simulink model "Record_Test"  (R2020a)
settings: Solver=VariableStepAuto  StartTime=0.0  StopTime=10  RelTol=1e-3
libraries: dspstat3 x3, audiosources x1, simulink x1, dspfdesign x1, dspvision x1, audiomeasurements x1
settings Model: Creator=Emil  LastModifiedBy=Emil

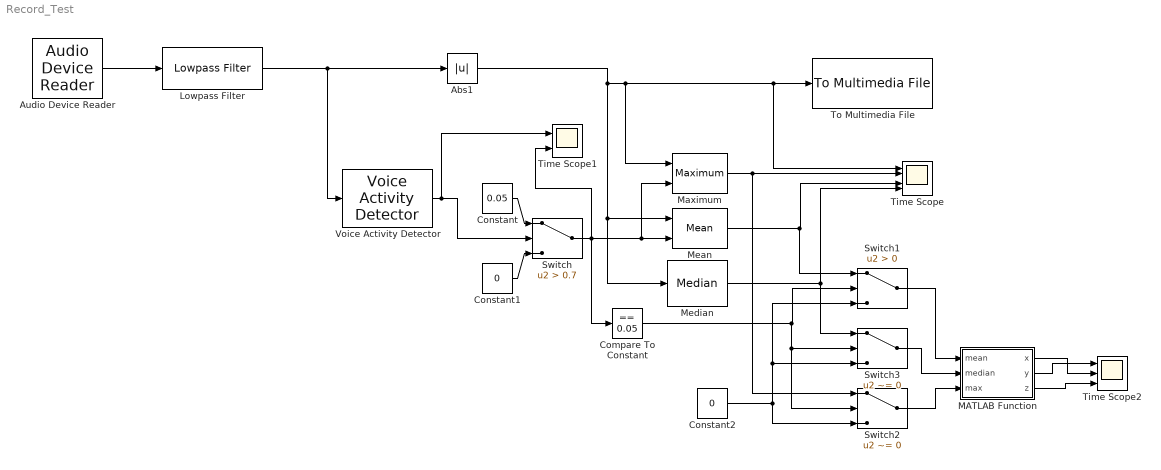
== system Record_Test ==
  Abs1 : Abs
  Audio Device Reader : audiosources/Audio Device Reader  Driver=DirectSound  Device=Default  SampleRate=44100  NumChannels=1  SamplesPerFrame=1024  BitDepth=16-bit integer  NumBuffers=10  DefaultInputChannelMapping=on  InputChannelMapping=1:2  OutputNumOverrunSamples=off  OutputDataType=double  DriverIdx=1  DeviceWarnFlag=''
      settings: SourceProductBaseCode=AU
  Compare To Constant : simulink/Logic and Bit Operations/Compare To Constant  relop===  const=0.05  OutDataTypeStr=boolean
  Constant : Constant  Value=0.05
  Constant1 : Constant  Value=0
  Constant2 : Constant  Value=0
  Lowpass Filter : dspfdesign/Lowpass Filter  FilterType=FIR  DesignForMinimumOrder=on  FilterOrder=50  PassbandFrequency=2.2e3  StopbandFrequency=3e3  PassbandRipple=0.1  StopbandAttenuation=80  InheritSampleRate=off  SampleRate=44100  SimulateUsing=Interpreted execution  roundingMode=Floor  coeffsDataTypeStr=fixdt(1,16)
  MATLAB Function : MATLAB Function  TreatAsAtomicUnit=on
  Maximum : dspstat3/Maximum  operation=maximum  fcn=Running  indexBase=One  operateOver=Entire input  Dimension=1  InputProcessing=Columns as channels (frame based)  reset=Either edge  roiEnable=off  roiType=Rectangles  roiPortion=Entire ROI  roiOutput=Individual statistics for each ROI  roiFlag=off  roundingMode=Nearest  overflowMode=off  accumDataTypeStr=Inherit: Same as product output  accumLastDataTypeStr=Inherit: Same as product output
  Mean : dspstat3/Mean  run=on  InputProcessing=Columns as channels (frame based)  reset_popup=Either edge  directionMode=Entire input  dimension=1  roiEnable=off  roiType=Rectangles  roiPortion=Entire ROI  roiOutput=Individual statistics for each ROI  roiFlag=off  roundingMode=Nearest  overflowMode=off  outputDataTypeStr=Inherit: Same as accumulator  outputMin=[1]  outputMax=[]  outputLastDataTypeStr=Inherit: Same as accumulator
  Median : dspstat3/Median  sortAlg=Quick sort  directionMode=Entire input  dimension=1  roundingMode=Floor  overflowMode=off  accumDataTypeStr=Inherit: Same as product output  accumLastDataTypeStr=Inherit: Same as product output  outputDataTypeStr=Inherit: Same as accumulator  outputMin=[0.06]  outputMax=[]  outputLastDataTypeStr=Inherit: Same as accumulator
      settings: SourceProductBaseCode=DS  allowOverrides=off
  Switch : Switch  Criteria=u2 > Threshold  Threshold=0.7
  Switch1 : Switch  Criteria=u2 > Threshold
  Switch2 : Switch  Criteria=u2 ~= 0
  Switch3 : Switch  Criteria=u2 ~= 0
  Time Scope : Scope  NumInputPorts=5
  Time Scope1 : Scope  NumInputPorts=2
  Time Scope2 : Scope  NumInputPorts=3
  To Multimedia File : dspvision/To Multimedia File  outputFilename=Test.wav  streamSelection=Audio only  videoCompressor=None (uncompressed)  audioCompressor=None (uncompressed)  imagePorts=Separate color signals  fileType=WAV  audioDatatype=16-bit integer  fourcc=RGB  videoQuality=75  mj2000CompFactor=10
  Voice Activity Detector : audiomeasurements/Voice Activity Detector  InputDomain=Time  Window=Hann  SidelobeAttenuation=60  InheritFFTLength=on  FFTLength=1024  SilenceToSpeechProbabilityPort=off  SilenceToSpeechProbability=0.2  SpeechToSilenceProbabilityPort=off  SpeechToSilenceProbability=0.1  OutputNoiseVariance=off  SimulateUsing=Code generation
      settings: SourceProductBaseCode=AU
  wires:
  Mean/1 -> Switch1/1, Time Scope/4
  Constant/1 -> Switch/1
  Constant1/1 -> Switch/3
  Voice Activity Detector/1 -> Time Scope1/1, Switch/2
  Switch/1 -> Time Scope1/2, Compare To Constant/1, Maximum/2, Mean/2
  Maximum/1 -> Switch2/1, Time Scope/2
  Median/1 -> Switch3/1, Time Scope/5
  Compare To Constant/1 -> Switch2/2, Switch3/2, Switch1/2
  Constant2/1 -> Switch1/3, Switch3/3, Switch2/3
  Switch1/1 -> MATLAB Function/1(mean)
  Switch3/1 -> MATLAB Function/2(median)
  Switch2/1 -> MATLAB Function/3(max)
  Audio Device Reader/1 -> Lowpass Filter/1
  MATLAB Function/2(y) -> Time Scope2/1
  MATLAB Function/1(x) -> Time Scope2/2
  MATLAB Function/3(z) -> Time Scope2/3
  Lowpass Filter/1 -> Abs1/1, Voice Activity Detector/1
  Abs1/1 -> Median/1, Mean/1, Time Scope/1, To Multimedia File/1, Maximum/1

== matlab function Record_Test/MATLAB Function ==
  data: x output; mean input; y output; median input; max input; z output


function [x,y,z] = fcn(mean,median,max)
hej = [0]
if mean ~= 0
   hej = [hej mean];
else
   test = mean(hej);
   i = 0;
   hej = (1000);
end

if(median ~= 0)
   
end
if(max ~= 0)
    
end
x = test;
y = median;
z = max;
